simulink model "test_branch2_gen"  (Simulink 7.7)
settings: Solver=FixedStepDiscrete  StartTime=0.0  StopTime=10000.0  FixedStep=1  RelTol=1e-3
libraries: SimpleModeling x3
settings Model: Creator=iris  LastModifiedBy=iris
settings DataIOCC: LimitDataPoints=off  SaveFormat=StructureWithTime  SignalLogging=off
settings OptimizationCC: BlockReduction=off  ConditionallyExecuteInputs=off  InlineParams=on
settings DebuggingCC: AlgebraicLoopMsg=error
settings HardwareCC: ProdHWDeviceType=ASIC/FPGA->ASIC/FPGA  TargetIntDivRoundTo=Zero  TargetEndianess=LittleEndian  TargetHWDeviceType=MATLAB Host  ProdEqTarget=off

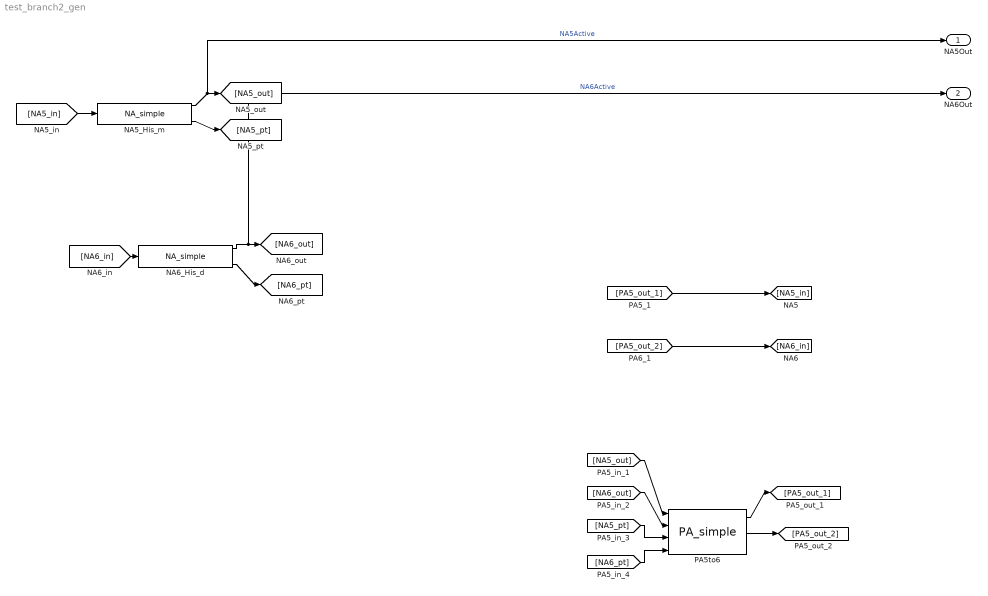
== system test_branch2_gen ==
  NA5_His_m : SimpleModeling/NA_simple  SystemSampleTime=-1  TERP_defs=320  TRRP_def=120  Trest_def=700  TERP_s=320  TRRP_s=120  Trest_s=700  Terp_min=150  Terp_max=300
  NA6_His_d : SimpleModeling/NA_simple  SystemSampleTime=-1  TERP_defs=320  TRRP_def=120  Trest_def=9999  TERP_s=320  TRRP_s=120  Trest_s=9999  Terp_min=150  Terp_max=300
  PA5to6 : SimpleModeling/PA_simple  SystemSampleTime=-1  min_path_par=20  bck_param=20  forw_param=20
  NA5Out : Outport
  NA6Out : Outport  Port=2
  wires:
  NA5_His_m/1 -> [NA5_out], NA5Out/1  "NA5Active"
  NA5_His_m/3 -> [NA5_pt]
  NA6_His_d/1 -> [NA6_out], NA6Out/1  "NA6Active"
  NA6_His_d/3 -> [NA6_pt]
  [NA6_in] -> NA6_His_d/1
  PA5to6/1 -> [PA5_out_1]
  PA5to6/2 -> [PA5_out_2]
  [NA5_out] -> PA5to6/1
  [NA6_out] -> PA5to6/2
  [NA5_pt] -> PA5to6/3
  [NA6_pt] -> PA5to6/4
  [PA5_out_1] -> [NA5_in]
  [NA5_in] -> NA5_His_m/1
  [PA5_out_2] -> [NA6_in]
